simulink model "SimulatorUnityConnection2"  (R2022b)
settings: configuration reference "WheelSimConfiguration" (kept outside this file)
undefined symbols (not defined in the file): simulator
libraries: slrealtimeloglib x4
settings Model: SimulationMode=external  Creator=MOSA  LastModifiedBy=MOSA
settings ConfigSetRef: SourceName=WheelSimConfiguration  SourceLocation=Base Workspace

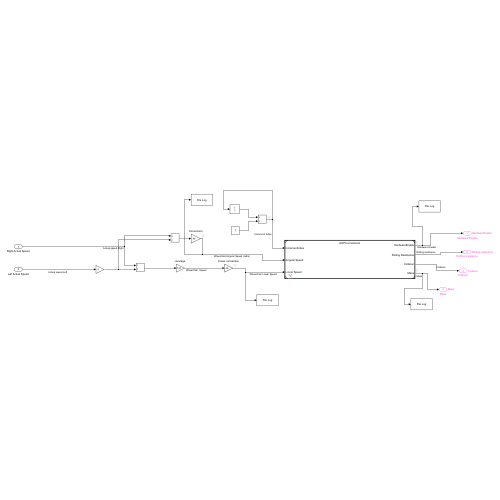
[thumbnail: Simulink's stored preview of the top-level diagram]
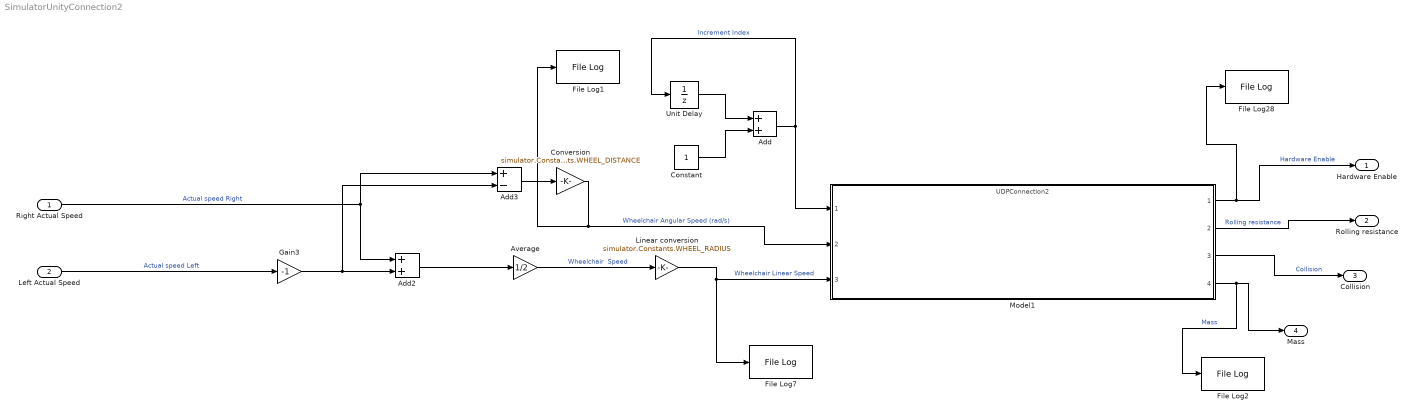
== system SimulatorUnityConnection2 ==
  Right Actual Speed : Inport
  Left Actual Speed : Inport  Port=2
  Add : Sum
  Add2 : Sum
  Add3 : Sum  Inputs=+-
  Average : Gain  Gain=1/2
  Constant : Constant
  Conversion : Gain  Gain=simulator.Constants.WHEEL_RADIUS/simulator.Constants.WHEEL_DISTANCE
  File Log{1..2,7,28} (4 alike) : slrealtimeloglib/File Log  decimation=1  inputProcessing=Elements as channels (sample based)
  Gain3 : Gain  Gain=-1
  Linear conversion : Gain  Gain=simulator.Constants.WHEEL_RADIUS
  Model1 : ModelReference  ModelNameDialog=UDPConnection2.slx  SimulationMode=Normal  ModelReferenceVersion=1.79
  Unit Delay : UnitDelay  SampleTime=-1  HasFrameUpgradeWarning=on
  Hardware Enable : Outport  SignalName=HardwareEnable
  Rolling resistance : Outport  Port=2  SignalName=Rolling resistance
  Collision : Outport  Port=3  SignalName=Collision
  Mass : Outport  Port=4  SignalName=Mass
  wires:
  Add2/1 -> Average/1
  Add3/1 -> Conversion/1
  Model1/2 -> Rolling resistance/1  "Rolling resistance"
  Model1/3 -> Collision/1  "Collision"
  Gain3/1 -> Add3/2, Add2/2
  Right Actual Speed/1 -> Add3/1, Add2/1  "Actual speed Right"
  Left Actual Speed/1 -> Gain3/1  "Actual speed Left"
  Linear conversion/1 -> File Log7/1, Model1/3  "Wheelchair Linear Speed"
  Average/1 -> Linear conversion/1  "Wheelchair  Speed"
  Conversion/1 -> Model1/2, File Log1/1  "Wheelchair Angular Speed (rad/s)"
  Model1/1 -> File Log28/1, Hardware Enable/1  "Hardware Enable"
  Add/1 -> Model1/1, Unit Delay/1  "Increment Index"
  Constant/1 -> Add/2
  Unit Delay/1 -> Add/1
  Model1/4 -> File Log2/1, Mass/1  "Mass"
